simulink model "FDM_TEST"  (R2017b)
settings: Solver=FixedStepDiscrete  StartTime=0.0  StopTime=10.0  RelTol=1e-3
libraries: commanapbnd3 x2
settings Model: Creator=admin  LastModifiedBy=admin

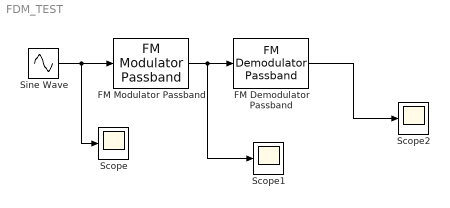
== system FDM_TEST ==
  FM Demodulator Passband : commanapbnd3/FM Demodulator Passband  Fc=8  Ph=0  Kc=500  Ho=80
      settings: SourceProductName=Communications System Toolbox  SourceProductBaseCode=CM
  FM Modulator Passband : commanapbnd3/FM Modulator Passband  Fc=8  Ph=0  Kc=5
      settings: SourceProductName=Communications System Toolbox  SourceProductBaseCode=CM
  Scope : Scope
  Scope1 : Scope
  Scope2 : Scope
  Sine Wave : Sin  Frequency=6  SampleTime=0.01
  wires:
  Sine Wave/1 -> Scope/1, FM Modulator Passband/1
  FM Modulator Passband/1 -> Scope1/1, FM Demodulator Passband/1
  FM Demodulator Passband/1 -> Scope2/1
